simulink model "subsystem_mask__test"  (Simulink 8.4)
settings: Solver=ode45  StartTime=0.0  StopTime=10.0  RelTol=1e-3
libraries: simulink x1
settings Model: Creator=arnaud  LastModifiedBy=arnaud
settings DataIOCC: SaveFormat=StructureWithTime

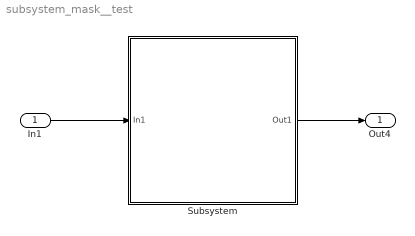
== system subsystem_mask__test ==
  In1 : Inport  PortDimensions=1
  Subsystem : Subsystem  TreatAsAtomicUnit=on
      mask Display: image('plane.jpg')
  Out4 : Outport
  wires:
  In1/1 -> Subsystem/1(In1)
  Subsystem/1(Out1) -> Out4/1

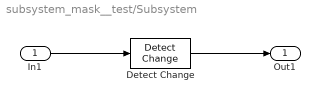
== system subsystem_mask__test/Subsystem ==
  In1 : Inport
  Detect Change : simulink/Logic and Bit Operations/Detect Change  vinit=0  InputProcessing=Inherited  OutDataTypeStr=boolean
  Out1 : Outport
  wires:
  In1/1 -> Detect Change/1
  Detect Change/1 -> Out1/1
